simulink model "find6DOFSnell_th"  (R2018b)
settings: Solver=ode8  StartTime=0.0  StopTime=4446  FixedStep=1  RelTol=1e-3
values from neighbouring files (symbols this model uses):
  GFC2Bottom = calculateRotationMatrix(botEulerAngles_rad(1),botEulerAngles_rad(2),botEulerAngles_rad(3))    [find6DoFSBFGS_init.m]
  GFC2Side = calculateRotationMatrix(sideEulerAngles_rad(1),sideEulerAngles_rad(2),sideEulerAngles_rad(3))    [find6DoFSBFGS_init.m]
  GFC2Slant = calculateRotationMatrix(slantEulerAngles_rad(1),slantEulerAngles_rad(2),slantEulerAngles_rad(3))    [find6DoFSBFGS_init.m]
undefined symbols (not defined in the file or in its folder): Find6DOFSnell, find6DOFSnell_cl, getVal
libraries: FindUnitVectorComponents_ul x4, rayTrace_ul x4, findEulerAngles_ul x1, findUnitVectors_ul x1, snellLeastSquaresPosition_ul x1
settings Model: Creator=mcobb  LastModifiedBy=MAE-NCSUCORE

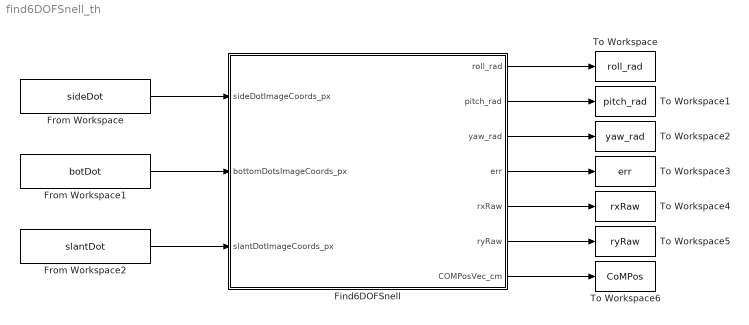
== system find6DOFSnell_th ==
  Find6DOFSnell : Subsystem  AncestorBlock=find6DOFSnell_cl/Find6DOFSnell  mask{imageDims_px=getVal('sideImageSize_px'), initialCoMPositionVec_cm=getVal('initCoMPosVec_cm'), indxOfRefVec=[1 1 1], glassThickness_cm=0.75*2.54, cameraFOVAngles_deg=getVal('cameraFOV_deg'), sideEulerAngles_deg=[0 89.2 89.5], sideCamPositionVec_cm=[10 39.5 67.5], sideCamDistToGlass_cm=2, botEulerAngles_deg=[0.2 179 180], botCamPositionVec_cm=[12 -2 22.5], botCamDistToGlass_cm=5, slantEulerAngles_deg=[0 133.9 180.6], slantCamPositionVec_cm=[-30.5 -2 26], slantCamDistToGlass_cm=7, sideSeparation_cm=getVal('sideDotSepDist_cm'), sidePositionVecBF_cm=[0.091 4.54 0.878], bottomASeparation_cm=getVal('botADotSepDist_cm'), botAPositionVecBF_cm=[2.48 0 -4.53], bottomBSeparation_cm=getVal('botBDotSepDist_cm'), botBPositionVecBG_cm=[-1 0 -4.64]}
      mask prompts: imageDims_px "Image Dimensions [rows, cols] [px]"; initialCoMPositionVec_cm "Initial CoM Position Vector [cm]"; indxOfRefVec "Indices of refraction, [air glass water]"; glassThickness_cm "Glass thickness [cm]"; cameraFOVAngles_deg "Field of View Angles [horiz, vert] [deg]"; sideEulerAngles_deg "Euler Angles [roll pitch yaw] [deg]"; sideCamPositionVec_cm "Position Vector [cm]"; sideCamDistToGlass_cm "Distance to Glass, [cm]"; botEulerAngles_deg "Euler Angles [roll pitch yaw]  [deg]"; botCamPositionVec_cm "Position Vector [cm]"; botCamDistToGlass_cm "Distance to Glass, [cm]"; slantEulerAngles_deg "Euler Angles [roll pitch yaw]  [deg]"; slantCamPositionVec_cm "Position Vec [cm]"; slantCamDistToGlass_cm "Distance to Glass, [cm]"; sideSeparation_cm "Separation Distance [cm]"; sidePositionVecBF_cm "Centroid Position in Body Frame [cm]"; bottomASeparation_cm "Separation Distance [cm]"; botAPositionVecBF_cm "Centroid Position in Body Frame [cm]"; bottomBSeparation_cm "Separation Distance [cm]"; botBPositionVecBG_cm "Centroid Position in Body Frame [cm]"
      mask init:
      | find6DOF_init
      mask DialogControl Container4 Prompt: Camera Properties
      mask DialogControl Container14 Prompt: Side Camera
      mask DialogControl Container17 Prompt: Bottom Camera
      mask DialogControl Container18 Prompt: Slant Camera
      mask DialogControl Container13 Prompt: Dot Properties
      mask DialogControl Container11 Prompt: Side Dots
      mask DialogControl Container12 Prompt: Bottom Dot Set A
      mask DialogControl Container15 Prompt: Bottom Dot Set B
      mask Display:
      | image('blockImage.png',[.2, .2, .6, .6],'on');
      | 
      | port_label('input',1,'Side')
      | port_label('input',2,'Bottom')
      | port_label('input',3,'Slant')
      | 
      | port_label('output',1,'roll_rad')
      | port_label('output',2,'pitch_rad')
      | port_label('output',3,'yaw_rad')
      | port_label('output',4,'err')
      | port_label('output',5,'rxRaw')
      | port_label('output',6,'ryRaw')
      | port_label('output',7,'CoMPosVec_cm')
      | 
      | text(0.5, 1, 'Snells Law - Resolve 6 DOF', 'horizontalAlignment', 'center', ...
      |   'verticalAlignment', 'top')
  From Workspace : FromWorkspace  VariableName=sideDot  SampleTime=0
  From Workspace1 : FromWorkspace  VariableName=botDot  SampleTime=0
  From Workspace2 : FromWorkspace  VariableName=slantDot  SampleTime=0
  To Workspace : ToWorkspace  VariableName=roll_rad  SampleTime=-1
  To Workspace1 : ToWorkspace  VariableName=pitch_rad  SampleTime=-1
  To Workspace2 : ToWorkspace  VariableName=yaw_rad  SampleTime=-1
  To Workspace3 : ToWorkspace  VariableName=err  SampleTime=-1
  To Workspace4 : ToWorkspace  VariableName=rxRaw  SampleTime=-1
  To Workspace5 : ToWorkspace  VariableName=ryRaw  SampleTime=-1
  To Workspace6 : ToWorkspace  VariableName=CoMPos  SampleTime=-1
  wires:
  Find6DOFSnell/1(roll_rad) -> To Workspace/1
  Find6DOFSnell/7(COMPosVec_cm) -> To Workspace6/1
  Find6DOFSnell/6(ryRaw) -> To Workspace5/1
  Find6DOFSnell/5(rxRaw) -> To Workspace4/1
  Find6DOFSnell/4(err) -> To Workspace3/1
  Find6DOFSnell/3(yaw_rad) -> To Workspace2/1
  Find6DOFSnell/2(pitch_rad) -> To Workspace1/1
  From Workspace2/1 -> Find6DOFSnell/3(slantDotImageCoords_px)
  From Workspace1/1 -> Find6DOFSnell/2(bottomDotsImageCoords_px)
  From Workspace/1 -> Find6DOFSnell/1(sideDotImageCoords_px)

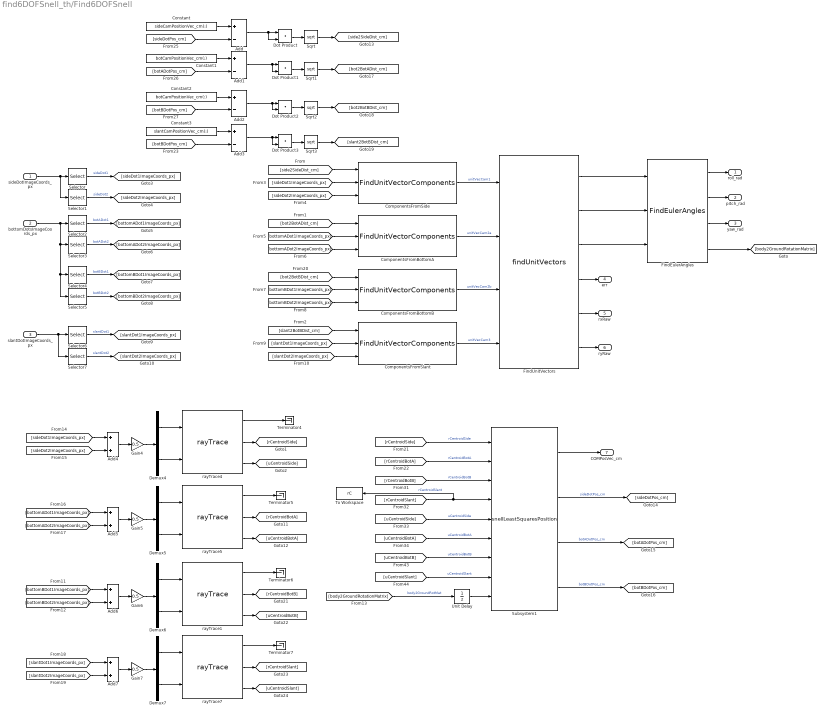
== system find6DOFSnell_th/Find6DOFSnell ==
  sideDotImageCoords_px : Inport
  bottomDotsImageCoords_px : Inport  Port=2
  slantDotImageCoords_px : Inport  Port=3
  Add{,1..3} (4 alike) : Sum  Inputs=+-
  Add{4..7} (4 alike) : Sum
  ComponentsFromBottomA : FindUnitVectorComponents_ul/FindUnitVectorComponents  cameraViewAngleVec_deg=cameraFOVAngles_deg  cam2GroundRotationMatrix=GFC2Bottom'  imageDimensions=imageDims_px
  ComponentsFromBottomB : FindUnitVectorComponents_ul/FindUnitVectorComponents  cameraViewAngleVec_deg=cameraFOVAngles_deg  cam2GroundRotationMatrix=GFC2Bottom'  imageDimensions=imageDims_px
  ComponentsFromSide : FindUnitVectorComponents_ul/FindUnitVectorComponents  cameraViewAngleVec_deg=cameraFOVAngles_deg  cam2GroundRotationMatrix=GFC2Side'  imageDimensions=imageDims_px
  ComponentsFromSlant : FindUnitVectorComponents_ul/FindUnitVectorComponents  cameraViewAngleVec_deg=cameraFOVAngles_deg  cam2GroundRotationMatrix=GFC2Slant'  imageDimensions=imageDims_px
  Constant : Constant  Value=sideCamPositionVec_cm(:)
  Constant1 : Constant  Value=botCamPositionVec_cm(:)
  Constant2 : Constant  Value=botCamPositionVec_cm(:)
  Constant3 : Constant  Value=slantCamPositionVec_cm(:)
  Demux{4..7} (4 alike) : Demux  Outputs=2
  Dot Product{,1..3} (4 alike) : DotProduct  InputSameDT=on  OutDataTypeStr=Inherit: Inherit via internal rule
  FindEulerAngles : findEulerAngles_ul/FindEulerAngles  SystemSampleTime=-1
  FindUnitVectors : findUnitVectors_ul/findUnitVectors  sideSeparation_cm=sideSeparation_cm  bottomASeparation_cm=bottomASeparation_cm  bottomBSeparation_cm=bottomBSeparation_cm  DSB=DSB  DBL=DBL
  Gain{4..7} (4 alike) : Gain  Gain=0.5
  Selector : Selector  InputPortWidth=4  IndexOptions=Index vector (dialog)  Indices=[1 2]  OutputSizes=1
  Selector1 : Selector  InputPortWidth=4  IndexOptions=Index vector (dialog)  Indices=[3 4]  OutputSizes=1
  Selector2 : Selector  InputPortWidth=8  IndexOptions=Index vector (dialog)  Indices=[1 2]  OutputSizes=1
  Selector3 : Selector  InputPortWidth=8  IndexOptions=Index vector (dialog)  Indices=[3 4]  OutputSizes=1
  Selector4 : Selector  InputPortWidth=8  IndexOptions=Index vector (dialog)  Indices=[5 6]  OutputSizes=1
  Selector5 : Selector  InputPortWidth=8  IndexOptions=Index vector (dialog)  Indices=[7 8]  OutputSizes=1
  Selector6 : Selector  InputPortWidth=4  IndexOptions=Index vector (dialog)  Indices=[1 2]  OutputSizes=1
  Selector7 : Selector  InputPortWidth=4  IndexOptions=Index vector (dialog)  Indices=[3 4]  OutputSizes=1
  Sqrt{,1..3} (4 alike) : Sqrt  SaturateOnIntegerOverflow=on
  Subsystem1 : snellLeastSquaresPosition_ul/snellLeastSquaresPosition  sideDotPosVec_cm=sidePositionVecBF_cm  botADotPosVec_cm=botAPositionVecBF_cm  botBDotPosVec_cm=botBPositionVecBG_cm
  Terminator{4..7} (4 alike) : Terminator
  To Workspace : ToWorkspace  VariableName=rC  SampleTime=-1
  Unit Delay : UnitDelay  InitialCondition=eye(3)  SampleTime=-1
  rayTrace1 : rayTrace_ul/rayTrace  camPosVec_cm=botCamPositionVec_cm  camEulAngles_deg=botEulerAngles_deg  dist2Glass_cm=botCamDistToGlass_cm  indOfRefVec=indxOfRefVec  glassPlane=1  glassThickness_cm=glassThickness_cm  imageDimsVec_px=imageDims_px  camFOV_deg=cameraFOVAngles_deg
  rayTrace4 : rayTrace_ul/rayTrace  camPosVec_cm=sideCamPositionVec_cm  camEulAngles_deg=sideEulerAngles_deg  dist2Glass_cm=sideCamDistToGlass_cm  indOfRefVec=indxOfRefVec  glassPlane=2  glassThickness_cm=glassThickness_cm  imageDimsVec_px=imageDims_px  camFOV_deg=cameraFOVAngles_deg
  rayTrace5 : rayTrace_ul/rayTrace  camPosVec_cm=botCamPositionVec_cm  camEulAngles_deg=botEulerAngles_deg  dist2Glass_cm=botCamDistToGlass_cm  indOfRefVec=indxOfRefVec  glassPlane=1  glassThickness_cm=glassThickness_cm  imageDimsVec_px=imageDims_px  camFOV_deg=cameraFOVAngles_deg
  rayTrace7 : rayTrace_ul/rayTrace  camPosVec_cm=slantCamPositionVec_cm  camEulAngles_deg=slantEulerAngles_deg  dist2Glass_cm=slantCamDistToGlass_cm  indOfRefVec=indxOfRefVec  glassPlane=1  glassThickness_cm=glassThickness_cm  imageDimsVec_px=imageDims_px  camFOV_deg=cameraFOVAngles_deg
  roll_rad : Outport  Unit=rad
  pitch_rad : Outport  Port=2  Unit=rad
  yaw_rad : Outport  Port=3  Unit=rad
  err : Outport  Port=4
  rxRaw : Outport  Port=5
  ryRaw : Outport  Port=6
  COMPosVec_cm : Outport  Port=7  Unit=rad
  wires:
  Unit Delay/1 -> Subsystem1/9
  Dot Product3/1 -> Sqrt3/1
  Dot Product2/1 -> Sqrt2/1
  Dot Product1/1 -> Sqrt1/1
  Dot Product/1 -> Sqrt/1
  Constant3/1 -> Add3/1
  Constant2/1 -> Add2/1
  Constant1/1 -> Add1/1
  [botBDotPos_cm] -> Add3/2
  [botBDotPos_cm] -> Add2/2
  [botADotPos_cm] -> Add1/2
  Sqrt3/1 -> [slant2BotBDist_cm]
  Sqrt2/1 -> [bot2BotBDist_cm]
  Sqrt1/1 -> [bot2BotADist_cm]
  Add3/1 -> Dot Product3/1, Dot Product3/2
  Add2/1 -> Dot Product2/1, Dot Product2/2
  Add1/1 -> Dot Product1/1, Dot Product1/2
  Sqrt/1 -> [side2SideDist_cm]
  Add/1 -> Dot Product/2, Dot Product/1
  [sideDotPos_cm] -> Add/2
  Constant/1 -> Add/1
  Subsystem1/4 -> [botBDotPos_cm]  "botBDotPos_cm"
  Subsystem1/3 -> [botADotPos_cm]  "botADotPos_cm"
  Subsystem1/2 -> [sideDotPos_cm]  "sideDotPos_cm"
  Subsystem1/1 -> COMPosVec_cm/1
  Demux5/2 -> rayTrace5/2
  [uCentroidSide] -> Subsystem1/5  "uCentroidSide"
  rayTrace1/3 -> [uCentroidBotB]
  [rCentroidBotB] -> Subsystem1/3  "rCentroidBotB"
  [body2GroundRotationMatrix] -> Unit Delay/1  "body2GroundRotMat"
  [rCentroidSide] -> Subsystem1/1  "rCentroidSide"
  [rCentroidBotA] -> Subsystem1/2  "rCentroidBotA"
  [rCentroidSlant] -> To Workspace/1, Subsystem1/4  "rCentroidSlant"
  rayTrace5/2 -> [rCentroidBotA]
  [uCentroidBotB] -> Subsystem1/7  "uCentroidBotB"
  [bottomBDot1ImageCoords_px] -> Add6/1
  rayTrace4/2 -> [rCentroidSide]
  Demux4/2 -> rayTrace4/2
  [uCentroidSlant] -> Subsystem1/8  "uCentroidSlant"
  rayTrace7/2 -> [rCentroidSlant]
  [bottomBDot2ImageCoords_px] -> Add6/2
  [slantDot1ImageCoords_px] -> Add7/1
  [bottomADot2ImageCoords_px] -> Add5/2
  Demux7/2 -> rayTrace7/2
  [sideDot2ImageCoords_px] -> Add4/2
  rayTrace7/1 -> Terminator7/1
  [uCentroidBotA] -> Subsystem1/6  "uCentroidBotA"
  Demux7/1 -> rayTrace7/1
  rayTrace7/3 -> [uCentroidSlant]
  [slantDot2ImageCoords_px] -> Add7/2
  Demux4/1 -> rayTrace4/1
  rayTrace4/1 -> Terminator4/1
  Demux5/1 -> rayTrace5/1
  Gain4/1 -> Demux4/1
  Gain5/1 -> Demux5/1
  Add5/1 -> Gain5/1
  Add6/1 -> Gain6/1
  [bottomADot1ImageCoords_px] -> Add5/1
  rayTrace4/3 -> [uCentroidSide]
  [sideDot1ImageCoords_px] -> Add4/1
  Add4/1 -> Gain4/1
  rayTrace1/2 -> [rCentroidBotB]
  Add7/1 -> Gain7/1
  rayTrace5/1 -> Terminator5/1
  Gain7/1 -> Demux7/1
  Gain6/1 -> Demux6/1
  Demux6/1 -> rayTrace1/1
  rayTrace1/1 -> Terminator6/1
  Demux6/2 -> rayTrace1/2
  rayTrace5/3 -> [uCentroidBotA]
  FindEulerAngles/4 -> [body2GroundRotationMatrix]
  FindUnitVectors/6 -> ryRaw/1
  FindUnitVectors/5 -> rxRaw/1
  Selector7/1 -> [slantDot2ImageCoords_px]  "slantDot2"
  slantDotImageCoords_px/1 -> Selector6/1, Selector7/1
  Selector6/1 -> [slantDot1ImageCoords_px]  "slantDot1"
  Selector5/1 -> [bottomBDot2ImageCoords_px]  "botBDot2"
  Selector4/1 -> [bottomBDot1ImageCoords_px]  "botBDot1"
  Selector3/1 -> [bottomADot2ImageCoords_px]  "botADot2"
  Selector2/1 -> [bottomADot1ImageCoords_px]  "botADot1"
  bottomDotsImageCoords_px/1 -> Selector2/1, Selector3/1, Selector4/1, Selector5/1
  sideDotImageCoords_px/1 -> Selector/1, Selector1/1
  Selector1/1 -> [sideDot2ImageCoords_px]  "sideDot2"
  Selector/1 -> [sideDot1ImageCoords_px]  "sideDot1"
  [bot2BotBDist_cm] -> ComponentsFromBottomB/1
  [slant2BotBDist_cm] -> ComponentsFromSlant/1
  [bot2BotADist_cm] -> ComponentsFromBottomA/1
  [side2SideDist_cm] -> ComponentsFromSide/1
  FindUnitVectors/4 -> err/1
  FindEulerAngles/3 -> yaw_rad/1
  FindEulerAngles/2 -> pitch_rad/1
  FindEulerAngles/1 -> roll_rad/1
  [slantDot2ImageCoords_px] -> ComponentsFromSlant/3
  [slantDot1ImageCoords_px] -> ComponentsFromSlant/2
  [bottomBDot2ImageCoords_px] -> ComponentsFromBottomB/3
  [bottomBDot1ImageCoords_px] -> ComponentsFromBottomB/2
  [bottomADot2ImageCoords_px] -> ComponentsFromBottomA/3
  [bottomADot1ImageCoords_px] -> ComponentsFromBottomA/2
  [sideDot2ImageCoords_px] -> ComponentsFromSide/3
  [sideDot1ImageCoords_px] -> ComponentsFromSide/2
  FindUnitVectors/3 -> FindEulerAngles/3
  FindUnitVectors/1 -> FindEulerAngles/1
  FindUnitVectors/2 -> FindEulerAngles/2
  ComponentsFromSlant/1 -> FindUnitVectors/4  "unitVecCam3"
  ComponentsFromBottomB/1 -> FindUnitVectors/3  "unitVecCam2b"
  ComponentsFromBottomA/1 -> FindUnitVectors/2  "unitVecCam2a"
  ComponentsFromSide/1 -> FindUnitVectors/1  "unitVecCam1"
